simulink model "BEST2021_keyboard_template"  (R2021a)
settings: Solver=ode23t  StartTime=0.0  StopTime=180.1  FixedStep=0.05  RelTol=1e-3  EnableMultiTasking=on
model workspace (MAT data in the model file):
  mapForSim.obsMap = [0 0 0 0 0 0 0 0 0 0 0 0 ... (40000 elements, 200x200)]
  mapForSim.scaleFactor = 28.5714285714
  mapForSim.simMap = robotics.BinaryOccupancyGrid
  mapForSim.simMap.Grid = [1 1 1 1 1 1 1 1 1 1 1 1 ... (40000 elements, 200x200)]
  mapForSim.simMap.SharedProperties = matlabshared.autonomous.internal.SharedMapProperties
  mapForSim.simMap.SharedProperties.Resolution = 28.5714285714
  mapForSim.simMap.SharedProperties.GridSize = [200 200]
  mapForSim.simMap.SharedProperties.XLocalLimits = [0 7]
  mapForSim.simMap.SharedProperties.YLocalLimits = [0 7]
  mapForSim.simMap.SharedProperties.XWorldLimits = [0 7]
  mapForSim.simMap.SharedProperties.YWorldLimits = [0 7]
  mapForSim.simMap.SharedProperties.Width = 7
  mapForSim.simMap.SharedProperties.Height = 7
  mapForSim.simMap.SharedProperties.LocalOriginInWorldInternal = [0 0]
  mapForSim.simMap.LayerName = 'binaryLayer'
  mapForSim.simMap.Index = matlabshared.autonomous.internal.CircularBufferIndex
  mapForSim.simMap.Index.Head = [1 1]
  mapForSim.simMap.Index.Size = [200 200]
  mapForSim.simMap.Index.NewRegions = [0 0 0 0]
  mapForSim.simMap.Index.DropEntireMap = 0
  mapForSim.simMap.Index.DropTwoRegions = [0 0]
  mapForSim.simMap.Buffer = matlabshared.autonomous.internal.CircularBuffer
  mapForSim.simMap.Buffer.ConstVal = 0
  mapForSim.simMap.Buffer.DataType = 'logical'
  mapForSim.simMap.Buffer.Index = matlabshared.autonomous.internal.CircularBufferIndex
  mapForSim.simMap.Buffer.Index.Head = [1 1]
  mapForSim.simMap.Buffer.Index.Size = [200 200]
  mapForSim.simMap.Buffer.Index.NewRegions = [0 0 0 0]
  mapForSim.simMap.Buffer.Index.DropEntireMap = 0
  mapForSim.simMap.Buffer.Index.DropTwoRegions = [0 0]
  mapForSim.simMap.Buffer.Buffer = [1 1 1 1 1 1 1 1 1 1 1 1 ... (40000 elements, 200x200)]
  mapForSim.simMap.Buffer.BufferSize = [200 200 1]
  mapForSim.simMap.DefaultValueInternal = 0
  mapForSim.simMap.DataSize = [200 200]
  mapForSim.simMap.GridLocationInWorld = [0 0]
  mapForSim.simMap.GridOriginInLocal = [0 0]
  mapForSim.simMap.LocalOriginInWorld = [0 0]
  mapForSim.simMap.Resolution = 28.5714285714
  mapForSim.simMap.GridSize = [200 200]
  mapForSim.simMap.XLocalLimits = [0 7]
  mapForSim.simMap.YLocalLimits = [0 7]
  mapForSim.simMap.XWorldLimits = [0 7]
  mapForSim.simMap.YWorldLimits = [0 7]
  mapForSim.simMap.Width = 7
  mapForSim.simMap.Height = 7
  mapForSim.simMap.LocalOriginInWorldInternal = [0 0]
  occGrid = robotics.BinaryOccupancyGrid
  occGrid.Grid = [1 1 1 1 1 1 1 1 1 1 1 1 ... (40000 elements, 200x200)]
  occGrid.SharedProperties = matlabshared.autonomous.internal.SharedMapProperties
  occGrid.SharedProperties.Resolution = 28.5714285714
  occGrid.SharedProperties.GridSize = [200 200]
  occGrid.SharedProperties.XLocalLimits = [0 7]
  occGrid.SharedProperties.YLocalLimits = [0 7]
  occGrid.SharedProperties.XWorldLimits = [0 7]
  occGrid.SharedProperties.YWorldLimits = [0 7]
  occGrid.SharedProperties.Width = 7
  occGrid.SharedProperties.Height = 7
  occGrid.SharedProperties.LocalOriginInWorldInternal = [0 0]
  occGrid.LayerName = 'binaryLayer'
  occGrid.Index = matlabshared.autonomous.internal.CircularBufferIndex
  occGrid.Index.Head = [1 1]
  occGrid.Index.Size = [200 200]
  occGrid.Index.NewRegions = [0 0 0 0]
  occGrid.Index.DropEntireMap = 0
  occGrid.Index.DropTwoRegions = [0 0]
  occGrid.Buffer = matlabshared.autonomous.internal.CircularBuffer
  occGrid.Buffer.ConstVal = 0
  occGrid.Buffer.DataType = 'logical'
  occGrid.Buffer.Index = matlabshared.autonomous.internal.CircularBufferIndex
  occGrid.Buffer.Index.Head = [1 1]
  occGrid.Buffer.Index.Size = [200 200]
  occGrid.Buffer.Index.NewRegions = [0 0 0 0]
  occGrid.Buffer.Index.DropEntireMap = 0
  occGrid.Buffer.Index.DropTwoRegions = [0 0]
  occGrid.Buffer.Buffer = [1 1 1 1 1 1 1 1 1 1 1 1 ... (40000 elements, 200x200)]
  occGrid.Buffer.BufferSize = [200 200 1]
  occGrid.DefaultValueInternal = 0
  occGrid.DataSize = [200 200]
  occGrid.GridLocationInWorld = [0 0]
  occGrid.GridOriginInLocal = [0 0]
  occGrid.LocalOriginInWorld = [0 0]
  occGrid.Resolution = 28.5714285714
  occGrid.GridSize = [200 200]
  occGrid.XLocalLimits = [0 7]
  occGrid.YLocalLimits = [0 7]
  occGrid.XWorldLimits = [0 7]
  occGrid.YWorldLimits = [0 7]
  occGrid.Width = 7
  occGrid.Height = 7
  occGrid.LocalOriginInWorldInternal = [0 0]
undefined symbols (not defined in the file): cellPose, FloorSurface, isoPoses, objectLevel, objectTypeArray, platformPoses, PlowSurface, Ref, RobotSurface, WallSurface, X, Y, Z
libraries: sm_lib x308, nesl_utility x151, simulink x76, RP_Simulator_Components x4
(part 1 of 15)
settings Model: EnablePacing=on  ExtModeTrigDuration=25  Creator=scastro  LastModifiedBy=josea
settings SolverCC: AlgebraicLoopSolver=LineSearch
settings DataIOCC: LimitDataPoints=on  SignalLogging=off  ReturnWorkspaceOutputs=off
settings OptimizationCC: DefaultParameterBehavior=Inlined  PassReuseOutputArgsAs=Individual arguments  MaxStackSize=64  EfficientTunableParamExpr=on
settings DebuggingCC: ReadBeforeWriteMsg=DisableAll  WriteAfterWriteMsg=DisableAll  WriteAfterReadMsg=DisableAll  MultiTaskDSMMsg=none  ParameterPrecisionLossMsg=none  ParameterTunabilityLossMsg=error  UnconnectedLineMsg=none  AllowSymbolicDim=off  SFUnexpectedBacktrackingDiag=warning  SFNoUnconditionalDefaultTransitionDiag=warning  SFExecutionAtInitializationDiag=none  SFMachineParentedDataDiag=warning  ArithmeticOperatorsInVariantConditions=warning
settings HardwareCC: ProdBitPerPointer=32  ProdBitPerSizeT=32  ProdBitPerPtrDiffT=32  ProdLargestAtomicInteger=Long  ProdLargestAtomicFloat=Double  ProdWordSize=32  ProdHWDeviceType=ARM Compatible->ARM Cortex
settings ModelReferenceCC: UpdateModelReferenceTargets=IfOutOfDate
settings SFSimCC: SFSimEcho=off  SimUseLocalCustomCode=off  MATLABDynamicMemAlloc=off  CustomCodeUndefinedFunction=UseInterfaceOnly
settings RTWCC: SystemTargetFile=ert.tlc  TemplateMakefile=ert_default_tmf  GenerateReport=on  RTWUseLocalCustomCode=off  Toolchain=GNU Tools for ARM Embedded Processors  IncludeHyperlinkInReport=on  LaunchReport=on  GenerateTraceInfo=on  GenerateTraceReport=on  GenerateTraceReportSl=on  GenerateTraceReportSf=on  GenerateTraceReportEml=on
settings CodeAppCC: ForceParamTrailComments=on  IgnoreCustomStorageClasses=off  OperatorAnnotations=on  SimulinkDataObjDesc=on  SFDataObjDesc=on  InsertBlockDesc=on
settings ERTTargetCC: ExtModeStaticAllocSize=2048  ERTCustomFileTemplate=example_file_process.tlc
settings ConfigComp: CovMetricSettings=dw  CovSaveCumulativeToWorkspaceVar=on  CovSaveSingleToWorkspaceVar=on  CovExternalEMLEnable=off  CovSFcnEnable=off
settings SimscapeCC: SimscapeNominalValues="[{\"value\":\"10\",\"unit\":\"V\"},{\"value\":\"1\",\"unit\":\"A\"},{\"value\":\"10\",\"unit\":\"N*m\"},{\"value\":\"10\",\"unit\":\"bar\"},{\"value\":\"100\",\"unit\":\"kJ/kg\"},{\"value\":\"1\",\"unit\":\"kW\"},{\"value\":\"300\",\"unit\":\"K\"},{\"value\":\"100\",\"unit\":\"cm^3/s\"},{\"value\":\"1\",\"unit\":\"kN\"},{\"value\":\"1\",\"unit\":\"g/cm^3\"},{\"value\":\"1\",\"unit\":\"l\"},{\"value\":\"1\",\"unit\":\"cm^2\"},{\"value\":\"60\",\"unit\":\"Hz\"}]"  SimscapeLogOpenViewer=on  SimscapeLogDataHistory=10000
settings ConfigurationSet: Description=SimMechanics 2G
settings DiagnosticsConfigSet: SimMechanicsRigidlyBoundBlock=none
settings ExplorerConfigSet: InternalSimMechanicsExplorerSettings="<ExplorerConfiguration><canonicalview>default</canonicalview><AnimationSetting><BasePlaybackSpeed>1.0</BasePlaybackSpeed><PlaybackSpeedFactor>1.0</PlaybackSpeedFactor></AnimationSetting><TilePanel><TileInfo><Tiles Columns=\"2\" Count=\"3\" Rows=\"2\"><Column Weight=\"0.5\"/><Column Weight=\"0.5\"/><Row Weight=\"0.6225\"/><Row Weight=\"0.3775\"/><Tile Height=\"1\" Width=\"2\" X=\"0\" Y=\"0\"/><Tile Height=\"1\" Width=\"1\" X=\"0\" Y=\"1\"/><Tile Height=\"1\" Width=\"1\" X=\"1\" Y=\"1\"/></Tiles></TileInfo><SceneInfo><SceneViewer><BGColor><R>0.60000002384185791</R><G>0.60000002384185791</G><B>0.60000002384185791</B></BGColor><Camera><DoPerspective>on</DoPerspective><Position><X>-2.5</X><Y>0</Y><Z>0.469999999999999973</Z></Position><Center><X>-1.56030737921409157</X><Y>0</Y><Z>0.12797985667433126</Z></Center><Up><X>0.342020143325668713</X><Y>0</Y><Z>0.939692620785908428</Z></Up><ViewLimDist>1</ViewLimDist><YLim>0.466307658154998583</YLim><XLim>0.693540120144815364</XLim></Camera></SceneViewer><SceneViewer><BGColor><R>0.60000002384185791</R><G>0.60000002384185791</G><B>0.60000002384185791</B></BGColor><Camera><DoPerspective>off</DoPerspective><Position><X>3.5332314785771386</X><Y>-3.3947402734829315</Y><Z>3.53231830664862745</Z></Position><Center><X>0.446325858412655041</X><Y>-0.728979182990680097</Y><Z>0.58226398573312621</Z></Center><Up><X>-0.344859316417843731</X><Y>0.487999196814355329</Y><Z>0.801828432888458731</Z></Up><ViewLimDist>1</ViewLimDist><YLim>3.17773372136945431</YLim><XLim>3.8699959231376031</XLim></Camera></SceneViewer><SceneViewer><BGColor><R>0.60000002384185791</R><G>0.60000002384185791</G><B>0.60000002384185791</B></BGColor><Camera><DoPerspective>off</DoPerspective><Position><X>-0.106931959652509123</X><Y>-0.225697807623169988</Y><Z>4.9870492424192383</Z></Position><Center><X>-0.106931959652509123</X><Y>-0.225697807623169988</Y><Z>0.219820364094227116</Z></Center><Up><X>0</X><Y>1</Y><Z>-0</Z></Up><ViewLimDist>1</ViewLimDist><YLim>4.50241434266635565</YLim><XLim>5.48325526245981365</XLim></Camera></SceneViewer></SceneInfo></TilePanel><MechEditorPanel><Cameras><Camera><Id>Camera1</Id><Value><Name>RobotView</Name><NativeCamera><PositionTrackingFeature>BEST_Robotics_2021_Game_Double_Click.BEST_2021_Robot.Body.RobotCamera.F</PositionTrackingFeature><CenterTrackingFeature>BEST_Robotics_2021_Game_Double_Click.BEST_2021_Robot.Body.RobotCamera.F</CenterTrackingFeature><UpVectorTrackingFeature>BEST_Robotics_2021_Game_Double_Click.BEST_2021_Robot.Body.RobotCamera.F</UpVectorTrackingFeature><CenterTrackingOrigin>off</CenterTrackingOrigin><CenterTrackingDirection>+X</CenterTrackingDirection><UpVectorTrackingDirection>+Z</UpVectorTrackingDirection></NativeCamera></Value></Camera></Cameras><GfxPanelCameraMap><MapElement CameraMLId=\"Camera1\" GfxPanelIndex=\"0\"/></GfxPanelCameraMap><VideoCreator><PlaybackSpeedRatio>1.0</PlaybackSpeedRatio><FrameRate>16</FrameRate><VideoFormat>Motion JPEG AVI</VideoFormat><FrameSize>auto</FrameSize></VideoCreator></MechEditorPanel></ExplorerConfiguration>"

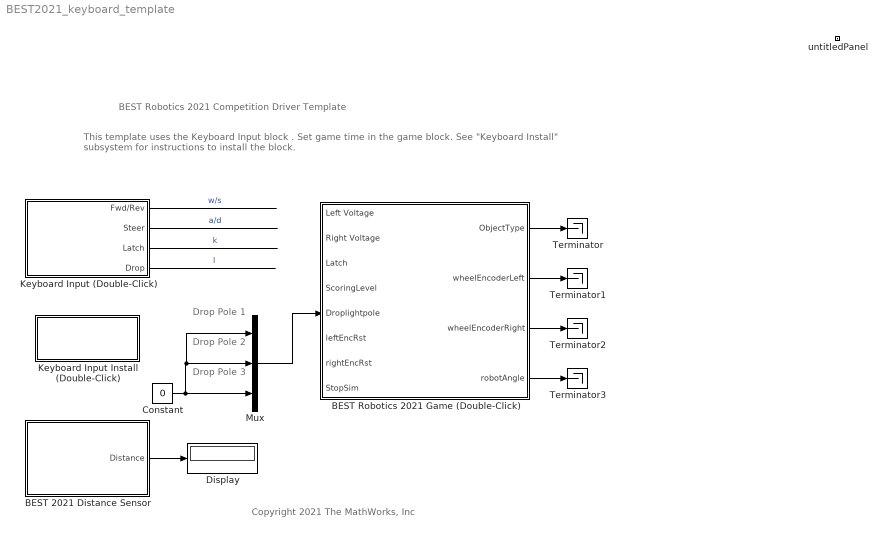
== system BEST2021_keyboard_template ==
  note: Copyright 2021 The MathWorks, Inc
  note: BEST Robotics 2021 Competition Driver Template
  note: This template uses the Keyboard Input block . Set game time in the game block.
      | See "Keyboard Install" subsystem for instructions to install the block.
  note: Drop Pole 1
  note: Drop Pole 2
  note: Drop Pole 3
  BEST 2021 Distance Sensor : Subsystem  mask(RP Distance Sensor){maxSenRange=10, minSenRange=0.02, senRes=0.01, sensOff=[0.25 0], sensOffDeg=0, sensorTs=0.1}
      mask prompts: maxSenRange "Maximum Range (m)"; minSenRange "Minimum Range (m)"; senRes "Resolution (m)"; sensOff "Sensor Position Offset X Y [m]"; sensOffDeg "Sensor Orientation Offset [deg]"; sensorTs "Sensor sample time [s]"
      mask help:
      | This block returns the distance to a nearby object such as walls and obstacles. Several sensor properties can be adjusted from the block mask, but default values can also be used.
      |
      | Sensor position and orientation are with respect to the robot center. Press the help button for more details on block parameters.
      mask Help: web('distance_sensor.htm')
      mask DialogControl senCont Prompt: Sensor Characteristics
      mask Display:
      | color('white');
      | plot([100,100,100,100]*1,[100,100,100,100]*1);
      | plot([100,100,100,100]*0,[100,100,100,100]*0);
      | image('ultrasonic_sensor.jpg','center')
      | color('blue');
      | 
      | text(99, 92, 'BEST 2021 Sensor', 'horizontalAlignment', 'right');
  BEST Robotics 2021 Game (Double-Click) : Subsystem  mask(RP BEST Robotics 2021 Challenge){gameTime=180, field=Practice 1, autoField=off, wheelBase=0.5, wheelRadius=0.1, robotColor=[0.5 0 0], wheelThickness=0.025, chassisThickness=0.05, wheelMass=1, chassisMass=1.5}
      mask prompts: gameTime "Game Time (s)"; field "Field Layout"; autoField "Finals"; wheelBase "Distance between wheels [m]"; wheelRadius "Wheel radius [m]"; robotColor "Color [R G B]"; wheelThickness "Wheel Thickness [m]"; chassisThickness "Chassis Thickness [m]"; wheelMass "Wheel Mass [kg]"; chassisMass "Chassis Mass [kg]"
      mask help:
      | This block contains a virtual game for the BEST Robotics 2021 competition. Please refere to the instructions provided by competition organizers for more information on game rules.
      |
      | Inputs:
      | Motor Voltages (Torque) [-127 to 127]
      | LatchObject (Pickup Object) [0 or 1]
      | RaiseObject (Floor or Dumpster) [0 or 1]
      | DropPole (Release pole) [0 or 1] Array of 3
      | Encoder Reset(normal operation or Reset) [0 or 1]
      |
      |
      | Outputs:
      | Object Type (See Game Rules) [0 ,1 , 2 ,3, 4, 5, 6, 7 or 8]
      | Sensors (See inside block for sensor properties and outputs)
      |
      | For MATLAB and Simulink related questions please email: roboticsarena@mathworks.com
      mask init:
      | autochoice=get_param(gcb,'autoField');
      | choice=get_param(gcb,'field');
      | time=get_param(gcb,'gameTime');
      | set_param(gcs,'StopTime',num2str(str2num(time)+0.1));
      | if strcmp(choice,'Practice 1')
      |   BEST2021GameConfigP1 
      | elseif strcmp(choice,'Practice 2')
      |   BEST2021GameConfigP2 
      | elseif strcmp(choice,'Practice 3')
      |   BEST2021GameConfigP3 
      | elseif strcmp(autochoice,"on")
      |    if strcmp(choice,'Phase 1 (Provided during competition)')
      |        BEST2021GameConfigFinals1
      |    elseif strcmp(choice,'Phase 2 (Provided during competition)')
      |      BEST2021GameConfigFinals2
      |    elseif strcmp(choice,'Phase 3 (Provided during competition)')
      |      BEST2021GameConfigFinals3
      |    elseif strcmp(choice,'Phase 4 (Provided during competition)')
      |      BEST2021GameConfigFinals4
      |    elseif strcmp(choice,'Phase 5 (Provided during competition)')
      |      BEST2021GameConfigFinals5
      |    elseif strcmp(choice,'Phase 6 (Provided during competition)')
      |      BEST2021GameConfigFinals6
      |    else
      |      BEST2021GameConfigFinals1
      |    end
      | elseif strcmp(choice,'Phase 1 (Provided during competition)')
      |   BEST2021GameConfig1
      | elseif strcmp(choice,'Phase 2 (Provided during competition)')
      |   BEST2021GameConfig2
      | elseif strcmp(choice,'Phase 3 (Provided during competition)')
      |   BEST2021GameConfig3
      | elseif strcmp(choice,'Phase 4 (Provided during competition)')
      |   BEST2021GameConfig4
      | elseif strcmp(choice,'Phase 5 (Provided during competition)')
      |   BEST2021GameConfig5
      | elseif strcmp(choice,'Phase 6 (Provided during competition)')
      |   BEST2021GameConfig6
      | else
      |   BEST2021GameConfig1 
      | end
      | 
      | block=gcb;
      | Arena.width=eval(get_param([block '/Arena'] ,'width'));
      | Arena.length=eval(get_param([block '/Arena'],'length'));
      | 
      | 
      | Arena.obj(1).status='on';
      | Arena.obj(1).position=eval(get_param([block '/Obstacles/Obstacle1'],'Pose'));
      | Arena.obj(1).width=eval(get_param([block '/Obstacles/Obstacle1'],'width'));
      | Arena.obj(1).length=eval(get_param([block '/Obstacles/Obstacle1'],'length'));
      | 
      | Arena.obj(2).status='on';
      | Arena.obj(2).position=eval(get_param([block '/Obstacles/Obstacle2'],'Pose'));
      | Arena.obj(2).width=eval(get_param([block '/Obstacles/Obstacle2'],'width'));
      | Arena.obj(2).length=eval(get_param([block '/Obstacles/Obstacle2'],'length'));
      | 
      | Arena.obj(3).status='on';
      | Arena.obj(3).position=eval(get_param([block '/Obstacles/Obstacle3'],'Pose'));
      | Arena.obj(3).width=eval(get_param([block '/Obstacles/Obstacle3'],'width'));
      | Arena.obj(3).length=eval(get_param([block '/Obstacles/Obstacle3'],'length'));
      | 
      | mapForSim=PlaygroundCreateSimMap(Arena,block);
      | ws=get_param(gcs,'modelworkspace');
      | 
      | assignin('base','mapForSim',mapForSim);
      | assignin('base','occGrid',mapForSim.simMap);
      mask TypeOptions field: Practice 1 | Practice 2 | Practice 3 | Phase 1 (Provided during competition) | Phase 2 (Provided during competition) | Phase 3 (Provided during competition) | Phase 4 (Provided during competition) | Phase 5 (Provided during competition) | Phase 6 (Provided during competition)
      mask TypeOptions wheelThickness: BEST 2021 Robot/wheelThickness
      mask TypeOptions chassisThickness: BEST 2021 Robot/chassisThickness
      mask TypeOptions wheelMass: BEST 2021 Robot/wheelMass
      mask TypeOptions chassisMass: BEST 2021 Robot/chassisMass
      mask DialogControl Container8 Prompt: Game Settings
      mask DialogControl Container4 Prompt: Robot settings
      mask DialogControl Container5 Prompt: Tab
      mask Display:
      | image('BEST2021environment.png')
      | port_label('input',1,'LeftMotor')
      | port_label('input',2,'RightMotor')
      | port_label('input',3,'LatchObject')
      | port_label('input',4,'RaiseObject')
      | port_label('input',5,'DropPole')
      | port_label('input',6,'EncoderLeftReset')
      | port_label('input',7,'EncoderRightReset')
      | port_label('input',8,'Stop Simulation')
      | port_label('output',1,'ObjectType')
      | port_label('output',2,'LeftEncoder')
      | port_label('output',3,'RightEncoder')
      | port_label('output',4,'RobotAngle')
  Constant : Constant  Value=0
  Display : Display
  Keyboard Input (Double-Click) : Subsystem
      mask Display: image('KeyboardIcon.PNG');
  Keyboard Input Install (Double-Click) : Subsystem
  Mux : Mux  Inputs=3
  Terminator{,1..3} (4 alike) : Terminator
  untitledPanel : Subsystem  Tag=HiddenForWebPanel  IsWebBlockPanel=on
  wires:
  BEST 2021 Distance Sensor/1(Distance) -> Display/1
  Keyboard Input (Double-Click)/2(Steer) -> ?  "a/d"
  Keyboard Input (Double-Click)/4(Drop) -> ?  "l"
  Keyboard Input (Double-Click)/1(Fwd/Rev) -> ?  "w/s"
  Constant/1 -> Mux/3, Mux/1, Mux/2
  Keyboard Input (Double-Click)/3(Latch) -> ?  "k"
  BEST Robotics 2021 Game (Double-Click)/2(wheelEncoderLeft) -> Terminator1/1
  BEST Robotics 2021 Game (Double-Click)/4(robotAngle) -> Terminator3/1
  BEST Robotics 2021 Game (Double-Click)/1(ObjectType) -> Terminator/1
  BEST Robotics 2021 Game (Double-Click)/3(wheelEncoderRight) -> Terminator2/1
  Mux/1 -> BEST Robotics 2021 Game (Double-Click)/5(Droplightpole)

== system BEST2021_keyboard_template/BEST 2021 Distance Sensor ==
  MATLAB System : MATLABSystem  System=LidarSensorRP  mapName=occGrid  sensorOffset=sensOff  scanAngles=sensOffDeg*pi/180  maxRange=maxSenRange
      mask Type: LidarSensorRP
      mask Display:
      | disp(['Lidar' char(10) 'Sensor']);
      | port_label('input',1,'pose');
      | port_label('output',1,'ranges');
  Mux : Mux  Inputs=3
  Quantizer : Quantizer  QuantizationInterval=senRes
  Rate Transition1 : RateTransition  OutPortSampleTime=sensorTs
  Saturation : Saturate  UpperLimit=maxSenRange  LowerLimit=minSenRange
  Distance : Outport  VectorParamsAs1DForOutWhenUnconnected=off
  wires:
  Rate Transition1/1 -> MATLAB System/1
  Saturation/1 -> Distance/1
  Quantizer/1 -> Saturation/1
  MATLAB System/1 -> Quantizer/1
  Mux/1 -> Rate Transition1/1
  [R1tPose] -> Mux/3
  [R1yPose] -> Mux/2
  [R1xPose] -> Mux/1

== system BEST2021_keyboard_template/BEST Robotics 2021 Game (Double-Click) ==
  note: DO NOT CHANGE THIS MODEL!
  Left Voltage : Inport
  Right Voltage : Inport  Port=2
  Latch : Inport  Port=3
  ScoringLevel : Inport  Port=4
  Droplightpole : Inport  Port=5
  leftEncRst : Inport  Port=6
  rightEncRst : Inport  Port=7
  StopSim : Inport  Port=8
  Arena : Subsystem  mask(RP Grid Arena){length=7, width=7}
      mask prompts: length "Arena length [m]"; width "Arena width [m]"
      mask help: This block is an arena for robots to operate within. This arena implements contact between one robot and the walls and also introduces a floor grid for better visualization. Connect to other robots within the library using the corresponding "Robot" and "Ref" ports.
      mask DialogControl Container5 Prompt: Arena dimensions
      mask Display:
      | image('BEST2021arena.png')
      | port_label('Lconn',1,'RP-Bus')
  BEST 2021 Robot : Subsystem  mask(RP Contact Tank Robot){robotId=1, wheelRadius=wheelRadius, wheelBase=wheelBase, wheelThickness=wheelThickness, chassisThickness=chassisThickness, startPose=[-2 0], choice=off, sensorTs=0.05, wheelMass=wheelMass, chassisMass=chassisMass, maxWheelTorque=2, wheelColor=[0.25 0.25 0.25], chassisColor=robotColor}
      mask prompts: robotId "Robot ID"; wheelRadius "Wheel Radius [m]"; wheelBase "Wheelbase [m]"; wheelThickness "Wheel Thickness [m]"; chassisThickness "Chassis Thickness [m]"; startPose "Start Position [m]"; choice "Reverse Start Position"; sensorTs "Sensor sample time [s]"; wheelMass "Wheel Mass [kg]"; chassisMass "Chassis Mass [kg]"; maxWheelTorque "Maximum wheel torque [N*m]"; wheelColor "Wheel Color"; chassisColor "Chassis Color"
      mask help:
      | This robot implements contact between the robot wheels and the floor of an arena. The stck-slip friction implemented using contact force libraries makes the robot behavior more realistic. The inputs to the robot are now motor torque, which is set using the Robotics Playground Motor blocks. The motor mappings are as follows:
      |
      | Motor 1 -> Left wheel motor torque
      | Motor 2 -> Right wheel motor torque
      mask init:
      | % This funciton is meant to add a sensor visualization from the components
      | % library to a robot 
      | %  Copyright 2018 The MathWorks, Inc.
      | 
      | % Disable the library link so all configurations can be saved with the
      | % model, otherwise it pulls from the library when model opens
      | blk=gcb;
      | set_param(blk,'LinkStatus','inactive');
      | 
      | % remove any existing visual blocks
      | 
      | subsystem = [blk '/Sensor Visuals'];
      | blocks = find_system(subsystem,'LookUnderMasks','all');
      | 
      | % Delete all previous blocks except the inport
      | for idx = 2:length(blocks)-1
      |     delete_block(blocks{idx})
      | end
      | 
      | % Delete all signals
      | while ~isempty(find_system(subsystem,'LookUnderMasks','all','FindAll','on','type','line'))
      |     lines = find_system(subsystem,'LookUnderMasks','all','FindAll','on','type','line');
      |     delete_line(lines(1))
      | end
      | % Set a position for the Physical connection port
      | pos1 = [140 100 180 140];
      | pos2 = [140 170 180 210];
      | 
      | set_param(strcat(subsystem,'/Robot'),'position',[140 60 180 80])
      | %%  Check for Distance sensors
      | 
      | sensors=find_system(bdroot,'MaskType','RP Distance Sensor');
      | 
      | if ~isempty(sensors)
      |     % Check for block with a matching Robot ID
      |     
      |     for idx=1:size(sensors,1)
      |             pos1 = pos1 + [60 0 60 0];
      |             pos2 = pos2 + [60 0 60 0];  
      | 
      |             % Get X Y sensor offsets
      |             xyOffset=get_param(sensors{idx},'sensOff');
      |             degOffset=get_param(sensors{idx},'sensOffDeg');
      |             
      |             % Add sensor visual and set parameters
      |             add_block('RP_Simulator_Components/US Visual',strcat(subsystem,'/US Visual ',num2str(idx)));
      |             set_param(strcat(subsystem,'/US Visual ',num2str(idx)),'position',pos1,'Orientation','down');
      |             set_param(strcat(subsystem,'/US Visual ',num2str(idx)),'pose',xyOffset,'angle',degOffset);
      |             add_line(subsystem,strcat('Robot','/Rconn1'),strcat('US Visual ',num2str(idx),'/LConn1'));                      
      |     end
      | end
      mask DialogControl KinContainer Prompt: Kinematics
      mask DialogControl DynamicsContainer Prompt: Dynamics
      mask DialogControl AppearanceContainer Prompt: Appearance
      mask Display:
      | image('BEST2020Robot.png')
      | port_label('Rconn',1,'RP-Bus')
  Compass Sensor : Subsystem  mask(RP Compass Sensor){sensorTs=0.1}
      mask prompts: sensorTs "Sensor sample time [s]"
      mask help: This sensor outputs the rotation in degrees as measured from the robot center relative to the world coordinate frame.
      mask Help: web('compass_sensor.htm')
      mask DialogControl senCont Prompt: Sensor Characteristics
      mask Display:
      | color('white');
      | plot([100,100,100,100]*1,[100,100,100,100]*1);
      | plot([100,100,100,100]*0,[100,100,100,100]*0);
      | image('Compass.png','center')
      | color('blue');
  Game Control : Subsystem
  Left Encoder : Subsystem  mask(RP Motor Encoder){rstChoice=Reset by external signal, ticks=180, detectDir=off, sensorTs=0.1}
      mask prompts: rstChoice "Reset option"; ticks "Ticks per rotation"; detectDir "Detect direction of rotation"; sensorTs "Sensor sample time [s]"
      mask help:
      | This block outputs the rotation in tick counts of an encoder conneted to the respective robot motor. You can set different sensor parameters from the mask or use the default settings.
      |
      | The most common use of motor encoders is to derive the position of an object. Start by converting the tick counts to revolutions of the motor shaft. You can later relate the revolutions of the motor shaft to more valuable robot information such as traveled distance by using robot dimensions like the wheel size.
      mask init:
      | blk=gcb;
      | 
      | switch get_param(blk,'rstChoice');
      | 
      |     case 'Reset by external signal'
      |         % Check for ground
      |      if strcmp(get_param([blk '/reset'],'BlockType'),'Ground')
      |             replace_block([blk '/reset'],'Ground','Inport','noprompt');
      |      end
      |     case 'No reset'
      |         % Check for inport
      |      if strcmp(get_param([blk '/reset'],'BlockType'),'Inport')
      |             replace_block([blk '/reset'],'Inport','Ground','noprompt')
      |      end
      | end
      mask Help: web('encoder_sensor.htm')
      mask TypeOptions rstChoice: No reset | Reset by external signal
      mask DialogControl ParameterGroupVar Prompt: Settings
      mask Display:
      | color('white');
      | plot([100,100,100,100]*1,[100,100,100,100]*1);
      | plot([100,100,100,100]*0,[100,100,100,100]*0);
      | image('encoder.jpg','center')
  Light poles : Subsystem
      mask Display: image('BEST2021lightpoles.png')
  Objects : Subsystem
      mask Display: image('BEST2021objects.png')
  Obstacles : Subsystem
      mask Display: image('obstacle-environment.png'); % Use "Edit Image" on toolstrip to change.
  Right Encoder : Subsystem  mask(RP Motor Encoder){rstChoice=Reset by external signal, ticks=180, detectDir=off, sensorTs=0.1}
      mask prompts: rstChoice "Reset option"; ticks "Ticks per rotation"; detectDir "Detect direction of rotation"; sensorTs "Sensor sample time [s]"
      mask help:
      | This block outputs the rotation in tick counts of an encoder conneted to the respective robot motor. You can set different sensor parameters from the mask or use the default settings.
      |
      | The most common use of motor encoders is to derive the position of an object. Start by converting the tick counts to revolutions of the motor shaft. You can later relate the revolutions of the motor shaft to more valuable robot information such as traveled distance by using robot dimensions like the wheel size.
      mask init: same as BEST2021_keyboard_template/BEST Robotics 2021 Game (Double-Click)/Left Encoder
      mask Help: web('encoder_sensor.htm')
      mask TypeOptions rstChoice: No reset | Reset by external signal
      mask DialogControl ParameterGroupVar Prompt: Settings
      mask Display:
      | color('white');
      | plot([100,100,100,100]*1,[100,100,100,100]*1);
      | plot([100,100,100,100]*0,[100,100,100,100]*0);
      | image('encoder.jpg','center')
  ObjectType : Outport
  wheelEncoderLeft : Outport  Port=2
  wheelEncoderRight : Outport  Port=3
  robotAngle : Outport  Port=4
  wires:
  Right Voltage/1 -> BEST 2021 Robot/2(In2)
  Left Voltage/1 -> BEST 2021 Robot/1(In1)
  Latch/1 -> Objects/1(Latch)
  Objects/1(ObjectType) -> ObjectType/1
  Right Encoder/1(Out1) -> wheelEncoderRight/1
  Left Encoder/1(Out1) -> wheelEncoderLeft/1
  BEST 2021 Robot/1(leftMotorW) -> Left Encoder/1(In1)
  BEST 2021 Robot/2(rightMotorW) -> Right Encoder/1(In1)
  BEST 2021 Robot/3(angle) -> Compass Sensor/1(angle)
  Compass Sensor/1(Distance) -> robotAngle/1
  Droplightpole/1 -> Light poles/2(Drop)
  ScoringLevel/1 -> Light poles/1("ScoreLevel "), Objects/2(ScoringLevel)
  leftEncRst/1 -> Left Encoder/2(reset)
  StopSim/1 -> Game Control/1(Stop)
  rightEncRst/1 -> Right Encoder/2(reset)
  connections:
  Light poles/LConn1 -- Obstacles/LConn1 -- Objects/LConn1 -- Arena/LConn1 -- BEST 2021 Robot/RConn1

== system BEST2021_keyboard_template/Keyboard Input (Double-Click) ==
  note: The operation of the keyboard input is CASE sensitive and only supports ONE KEY PRESSED at any given time
  note: ASCII Character Representation
  "\"A\" Key" : simulink/Logic and Bit Operations/Compare To Constant  relop===  const=97  OutDataTypeStr=boolean
  "\"D\" Key" : simulink/Logic and Bit Operations/Compare To Constant  relop===  const=100  OutDataTypeStr=boolean
  "\"K\" Key1" : simulink/Logic and Bit Operations/Compare To Constant  relop===  const=107  OutDataTypeStr=boolean
  "\"L\" Key1" : simulink/Logic and Bit Operations/Compare To Constant  relop===  const=108  OutDataTypeStr=boolean
  "\"S\" Key" : simulink/Logic and Bit Operations/Compare To Constant  relop===  const=115  OutDataTypeStr=boolean
  "\"W\" Key" : simulink/Logic and Bit Operations/Compare To Constant  relop===  const=119  OutDataTypeStr=boolean
  Add : Sum
  Add1 : Sum
  Data Type Conversion{,1..5} (6 alike) : DataTypeConversion  OutDataTypeStr=double
  Gain : Gain
  Gain1 : Gain  Gain=-1
  Gain2 : Gain
  Gain3 : Gain  Gain=-1
  Keyboard 1 : M-S-Function  FunctionName=sfun_keyboard_input_v1_2b  mask(Keyboard Input){}
      mask help: Keyboard Input
      mask Display: fprintf('Keyboard');
  Packet FIlter : Subsystem
  Product : Product
  Rate Transition : RateTransition
  Scope1 : Scope
  pulseLength (ms) : Constant  Value=60
  Fwd/Rev : Outport  VectorParamsAs1DForOutWhenUnconnected=off
  Steer : Outport  Port=2  VectorParamsAs1DForOutWhenUnconnected=off
  Latch : Outport  Port=3  VectorParamsAs1DForOutWhenUnconnected=off
  Drop : Outport  Port=4  VectorParamsAs1DForOutWhenUnconnected=off
  wires:
  "\"S\" Key"/1 -> Data Type Conversion1/1
  "\"W\" Key"/1 -> Data Type Conversion/1
  "\"A\" Key"/1 -> Data Type Conversion2/1
  "\"D\" Key"/1 -> Data Type Conversion3/1
  Gain/1 -> Scope1/1, Add/1
  Gain1/1 -> Add/2
  Gain2/1 -> Add1/1
  Gain3/1 -> Add1/2
  Product/1 -> "\"L\" Key1"/1, "\"K\" Key1"/1, "\"D\" Key"/1, "\"A\" Key"/1, "\"S\" Key"/1, "\"W\" Key"/1
  Add1/1 -> Steer/1
  Add/1 -> Fwd/Rev/1
  Data Type Conversion/1 -> Gain/1
  Data Type Conversion1/1 -> Gain1/1
  Data Type Conversion2/1 -> Gain2/1
  Data Type Conversion3/1 -> Gain3/1
  Keyboard 1/1 -> Rate Transition/1  "LastKey"
  Packet FIlter/1(Filtered) -> Product/2
  Keyboard 1/2 -> Packet FIlter/1(Ready)  "KeyIsPressed"
  Data Type Conversion5/1 -> Drop/1
  Data Type Conversion4/1 -> Latch/1
  "\"K\" Key1"/1 -> Data Type Conversion4/1
  "\"L\" Key1"/1 -> Data Type Conversion5/1
  Rate Transition/1 -> Product/1
  pulseLength (ms)/1 -> Packet FIlter/2(StretchLength)

== system BEST2021_keyboard_template/Keyboard Input Install (Double-Click) ==
  note: Alternatively download from here .
  note: 3. Add library to MATLAB
  note: 2. Find Simulink Keyboard Input V2
  note: Instructions to install Keyboard input block using Add-ons explorer
  note: 1. Open Add-On explorer

== system BEST2021_keyboard_template/untitledPanel ==
  Display : DisplayBlock  Tag=HiddenForWebPanel  PanelInfo="{\"panelId\":\"panelId-e4c80917-d596-452e-b167-d8f40ae9d3ef\",\"type\":\"panelChild\",\"version\":\"2019b\",\"zIndex\":1500020}"  LabelPosition=Hide  Format=short  Transparency=1
  Display1 : DisplayBlock  Tag=HiddenForWebPanel  PanelInfo="{\"panelId\":\"panelId-e4c80917-d596-452e-b167-d8f40ae9d3ef\",\"type\":\"panelChild\",\"version\":\"2019b\",\"zIndex\":1500008}"  LabelPosition=Hide  Format=short  Transparency=1
  Display2 : DisplayBlock  Tag=HiddenForWebPanel  PanelInfo="{\"panelId\":\"panelId-e4c80917-d596-452e-b167-d8f40ae9d3ef\",\"type\":\"panelChild\",\"version\":\"2019b\",\"zIndex\":1500022}"  LabelPosition=Hide  Format=short  Transparency=1
  Display3 : DisplayBlock  Tag=HiddenForWebPanel  PanelInfo="{\"panelId\":\"panelId-e4c80917-d596-452e-b167-d8f40ae9d3ef\",\"type\":\"panelChild\",\"version\":\"2019b\",\"zIndex\":1500024}"  LabelPosition=Hide  Format=short  Transparency=1
  Lamp : LampBlock  Tag=HiddenForWebPanel  PanelInfo="{\"panelId\":\"panelId-e4c80917-d596-452e-b167-d8f40ae9d3ef\",\"type\":\"panelChild\",\"version\":\"2019b\",\"zIndex\":1500002}"  LabelPosition=Hide
  Lamp1 : LampBlock  Tag=HiddenForWebPanel  PanelInfo="{\"panelId\":\"panelId-e4c80917-d596-452e-b167-d8f40ae9d3ef\",\"type\":\"panelChild\",\"version\":\"2019b\",\"zIndex\":1500004}"  LabelPosition=Hide
  Lamp2 : LampBlock  Tag=HiddenForWebPanel  PanelInfo="{\"panelId\":\"panelId-e4c80917-d596-452e-b167-d8f40ae9d3ef\",\"type\":\"panelChild\",\"version\":\"2019b\",\"zIndex\":1500010}"  LabelPosition=Hide
  Lamp3 : LampBlock  Tag=HiddenForWebPanel  PanelInfo="{\"panelId\":\"panelId-e4c80917-d596-452e-b167-d8f40ae9d3ef\",\"type\":\"panelChild\",\"version\":\"2019b\",\"zIndex\":1500012}"  LabelPosition=Hide
  Lamp4 : LampBlock  Tag=HiddenForWebPanel  PanelInfo="{\"panelId\":\"panelId-e4c80917-d596-452e-b167-d8f40ae9d3ef\",\"type\":\"panelChild\",\"version\":\"2019b\",\"zIndex\":1500014}"  LabelPosition=Hide
  Lamp5 : LampBlock  Tag=HiddenForWebPanel  PanelInfo="{\"panelId\":\"panelId-e4c80917-d596-452e-b167-d8f40ae9d3ef\",\"type\":\"panelChild\",\"version\":\"2019b\",\"zIndex\":1500016}"  LabelPosition=Hide
  Lamp6 : LampBlock  Tag=HiddenForWebPanel  PanelInfo="{\"panelId\":\"panelId-e4c80917-d596-452e-b167-d8f40ae9d3ef\",\"type\":\"panelChild\",\"version\":\"2019b\",\"zIndex\":1500018}"  LabelPosition=Hide
  panelInfo : PanelWebBlock  Tag=HiddenForWebPanel  PanelInfo="{\"compacted\":false,\"height\":336,\"isActiveTab\":true,\"labels\":{\"label0076574892\":{\"left\":\"16\",\"settings\":{\"backgroundColor\":\"rgba(0, 0, 0, 0)\",\"bold\":false,\"font\":\"Arial\",\"fontColor\":\"black\",\"fontSize\":0.67,\"italicized\":false,\"underlined\":false},\"text\":\"TrashPile\",\"top\":\"215\"},\"label2385704033\":{\"left\":\"81\",\"settings\":{\"backgroundColor\":\"rgba(0, 0, 0, 0)\",\"bold\":false,\"font\":\"Arial\",\"fontColor\":\"black\",\"fontSize\":0.67,\"italicized\":false,\"underlined\":false},\"text\":\"1\",\"top\":\"115\"},\"label2630059905\":{\"left\":\"80\",\"settings\":{\"backgroundColor\":\"rgba(0, 0, 0, 0)\",\"bold\":false,\"font\":\"Arial\",\"fontColor\":\"black\",\"fontSize\":0.67,\"italicized\":false,\"underlined\":false},\"text\":\"TOTAL SCORE\",\"top\":\"13\"},\"label3121914332\":{\"left\":\"26\",\"settings\":{\"backgroundColor\":\"rgba(0, 0, 0, 0)\",\"bold\":false,\"font\":\"Arial\",\"fontColor\":\"black\",\"fontSize\":0.67,\"italicized\":false,\"underlined\":false},\"text\":\"Reuse\",\"top\":\"295\"},\"label4085150698\":{\"left\":\"147\",\"settings\":{\"backgroundColor\":\"rgba(0, 0, 0, 0)\",\"bold\":false,\"font\":\"Arial\",\"fontColor\":\"black\",\"fontSize\":0.67,\"italicized\":false,\"underlined\":false},\"text\":\"Green\",\"top\":\"181\"},\"label4924794780\":{\"left\":\"14\",\"settings\":{\"backgroundColor\":\"rgba(0, 0, 0, 0)\",\"bold\":false,\"font\":\"Arial\",\"fontColor\":\"black\",\"fontSize\":0.67,\"italicized\":false,\"underlined\":false},\"text\":\"Light Poles\",\"top\":\"93\"},\"label5071279776\":{\"left\":\"19\",\"settings\":{\"backgroundColor\":\"rgba(0, 0, 0, 0)\",\"bold\":false,\"font\":\"Arial\",\"fontColor\":\"black\",\"fontSize\":0.67,\"italicized\":false,\"underlined\":false},\"text\":\"Recycle\",\"top\":\"255\"},\"label5509391692\":{\"left\":\"184\",\"settings\":{\"backgroundColor\":\"rgba(0, 0, 0, 0)\",\"bold\":false,\"font\":\"Arial\",\"fontColor\":\"black\",\"fontSize\":0.67,\"italicized\":false,\"underlined\":false},\"text\":\"Yellow\",\"top\":\"181\"},\"label5900019865\":{\"left\":\"151\",\"settings\":{\"backgroundColor\":\"rgba(0, 0, 0, 0)\",\"bold\":false,\"font\":\"Arial\",\"fontColor\":\"black\",\"fontSize\":0.67,\"italicized\":false,\"underlined\":false},\"text\":\"3\",\"top\":\"114\"},\"label6002516453\":{\"left\":\"24\",\"settings\":{\"backgroundColor\":\"rgba(0, 0, 0, 0)\",\"bold\":false,\"font\":\"Arial\",\"fontColor\":\"black\",\"fontSize\":0.67,\"italicized\":false,\"underlined\":false},\"text\":\"Fences\",\"top\":\"159\"},\"label7682775433\":{\"left\":\"116\",\"settings\":{\"backgroundColor\":\"rgba(0, 0, 0, 0)\",\"bold\":false,\"font\":\"Arial\",\"fontColor\":\"black\",\"fontSize\":0.67,\"italicized\":false,\"underlined\":false},\"text\":\"2\",\"top\":\"114\"},\"label9221373582\":{\"left\":\"78\",\"settings\":{\"backgroundColor\":\"rgba(0, 0, 0, 0)\",\"bold\":false,\"font\":\"Arial\",\"fontColor\":\"black\",\"fontSize\":0.67,\"italicized\":false,\"underlined\":false},\"text\":\"Blue\",\"top\":\"179\"},\"label9463609268\":{\"left\":\"116\",\"settings\":{\"backgroundColor\":\"rgba(0, 0, 0, 0)\",\"bold\":false,\"font\":\"Arial\",\"fontColor\":\"black\",\"fontSize\":0.67,\"italicized\":false,\"underlined\":false},\"text\":\"Red\",\"top\":\"180\"}},\"left\":633,\"name\":\"Panel\",\"panelId\":\"panelId-e4c80917-d596-452e-b167-d8f40ae9d3ef\",\"tabIndex\":0,\"tabbedSetId\":\"tabbedSet3938523500\",\"top\":20,\"type\":\"panel\",\"version\":\"2019b\",\"visible\":true,\"width\":232,\"zIndex\":1500002}"  PanelSnapshot=<binary blob, 20008 chars, not shown>

== system BEST2021_keyboard_template/BEST Robotics 2021 Game (Double-Click)/Arena ==
  Floor : Subsystem
  Mechanism Configuration : sm_lib/Utilities/Mechanism Configuration  UniformGravity=Constant  GravityVector=[0 0 -9.80665]  GravityVectorUnits=m/s^2  GravityUnits=m/s^2  LinearizationDelta=0.001  JointModeTransitionNonlinearIterations=2
  Simscape Bus : SimscapeBus  HierarchyStrings=WallSurface;FloorSurface;Ref
  Solver Configuration : nesl_utility/Solver Configuration  PhysicalDomain=network_engine_domain  SubClassName=solver  LeftPortType=input  RightPortType=generic  Tones=[]  Harmonics=[]  SimulateNoise=off  Profile=off  UseLocalSampling=off  EnableSwitchedLinearOptims=on  FrequencyDomain=off  UseCCode=off  RelTol=0.001  AbsTol=1e-06  MinStep=1e-09  ToWorkspace=off  RevertToSquareIcSolve=off  NumHomotopyIterations=100  PhasorMode=off  PhasorModeNumHarmonics=1  DoDC=off  ResidualTolerance=1e-08  UseLocalSolver=off  LocalSolverChoice=NE_BACKWARD_EULER_ADVANCER  LocalSolverSampleTime=0.0002  DoFixedCost=off  MaxNonlinIter=10  MaxModeIter=2  ComputeImpulses=off  ImpulseIterations=2  LinearAlgebra=Sparse  EquationFormulation=NE_TIME_EF  DelaysMemoryBudget=1024  AutomaticFiltering=off  FilteringTimeConstant=0.001  PartitionStorageMethod=AS_NEEDED  PartitionMemoryBudget=1024  PartitionMethod=FAST
      settings: SourceProductBaseCode=PW,SS
  World Frame : sm_lib/Frames and Transforms/World Frame
  RP-Bus : PMIOPort  Side=Left
  connections:
  World Frame/RConn1 -- Floor/RConn1 -- Mechanism Configuration/RConn1 -- Simscape Bus/LConn3 -- Solver Configuration/RConn1
  Simscape Bus/RConn1 -- RP-Bus/RConn1
  Simscape Bus/LConn2 -- Floor/LConn1
